simulink model "Problem1"  (R2020a)
settings: Solver=VariableStepAuto  StartTime=0.0  StopTime=10.0  RelTol=1e-3
settings Model: Creator=Shreyas  LastModifiedBy=Shreyas

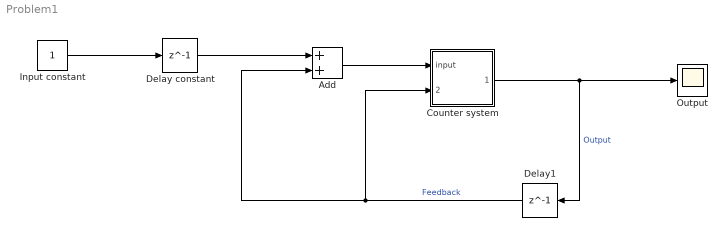
== system Problem1 ==
  Add : Sum
  Counter system : Stateflow chart  TreatAsAtomicUnit=on
  Delay constant : Delay  DelayLength=1  InitialCondition=0  UseCircularBuffer=on
  Delay1 : Delay  DelayLength=1  InitialCondition=0
  Input constant : Constant
  Output : Scope
  wires:
  Input constant/1 -> Delay constant/1
  Add/1 -> Counter system/1(input)
  Delay1/1 -> Add/2, Counter system/2(feedback)  "Feedback"
  Counter system/1(output) -> Output/1, Delay1/1  "Output"
  Delay constant/1 -> Add/1

== stateflow chart Problem1/Counter system ==
  (default) -> (junction 1) : % switch
  (junction 1) -> (junction 6) [order 1] : [feedback >= 5]
  (junction 1) -> (junction 4) [order 2] : {output = input;}
  (junction 6) -> (junction 8) : {output = 0;}
  (junction 8) -> (junction 4)
  (junction 4) -> (junction 11)
  data: input input; feedback input; output output
